simulink model "Practica3seminario"  (R2017b)
settings: Solver=VariableStepAuto  StartTime=0.0  StopTime=15  MaxStep=.01  RelTol=1e-3
settings Model: Creator=Charles  LastModifiedBy=Charles

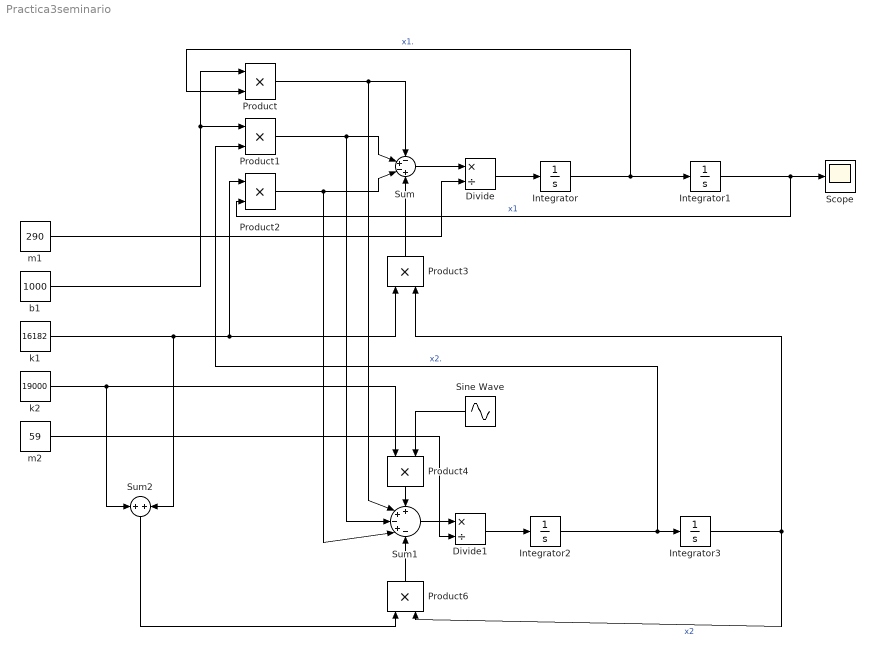
== system Practica3seminario ==
  Divide : Product  Inputs=*/
  Divide1 : Product  Inputs=*/
  Integrator{,1..3} (4 alike) : Integrator
  Product{,1..4,6} (6 alike) : Product
  Scope : Scope
  Sine Wave : Sin  Amplitude=.05  Frequency=.5*pi  SampleTime=0
  Sum : Sum  Inputs=-+-+
  Sum1 : Sum  Inputs=++-+-
  Sum2 : Sum
  "b1 " : Constant  Value=1000
  "k1 " : Constant  Value=16182
  k2 : Constant  Value=19000
  m1 : Constant  Value=290
  m2 : Constant  Value=59
  wires:
  Integrator/1 -> Integrator1/1, Product/2  "x1."
  Integrator1/1 -> Product2/2, Scope/1  "x1"
  Integrator2/1 -> Product1/2, Integrator3/1  "x2."
  Integrator3/1 -> Product6/2, Product3/2  "x2"
  Divide/1 -> Integrator/1
  Sum/1 -> Divide/1
  m1/1 -> Divide/2
  Divide1/1 -> Integrator2/1
  Sum1/1 -> Divide1/1
  m2/1 -> Divide1/2
  Product/1 -> Sum1/2, Sum/1
  "b1 "/1 -> Product1/1, Product/1
  Product1/1 -> Sum1/3, Sum/2
  Product2/1 -> Sum1/4, Sum/3
  "k1 "/1 -> Sum2/2, Product3/1, Product2/1
  Product3/1 -> Sum/4
  Product4/1 -> Sum1/1
  k2/1 -> Sum2/1, Product4/1
  Sine Wave/1 -> Product4/2
  Product6/1 -> Sum1/5
  Sum2/1 -> Product6/1
